simulink model "key_com_motor_ctrl"  (R2021a)
settings: configuration reference "f2_ctrl_config" (kept outside this file)
settings Model: DataDictionary=motor_data.sldd  Creator=Litao  LastModifiedBy=Litao
settings ConfigSetRef: SourceName=f2_ctrl_config

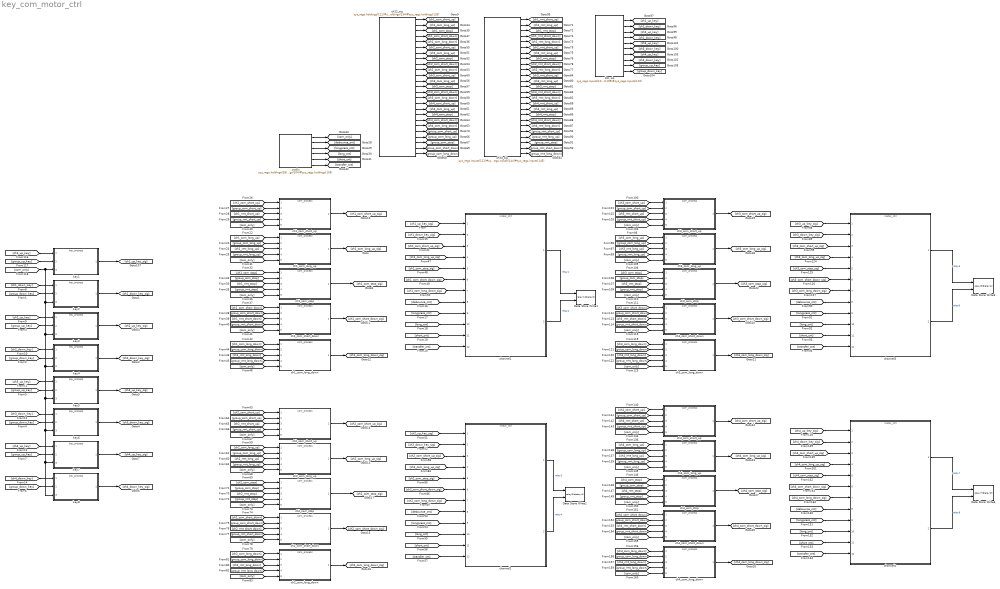
== system key_com_motor_ctrl ==
  Data Store Write1 : DataStoreWrite  DataStoreName=relay  DataStoreElements=relay(1)#relay(2)  IndexOptions=Index vector (dialog)  Indices=1  OutputSizes=1
  Data Store Write2 : DataStoreWrite  DataStoreName=relay  DataStoreElements=relay(3)#relay(4)  IndexOptions=Index vector (dialog)  Indices=1  OutputSizes=1
  Data Store Write3 : DataStoreWrite  DataStoreName=relay  DataStoreElements=relay(5)#relay(6)  IndexOptions=Index vector (dialog)  Indices=1  OutputSizes=1
  Data Store Write4 : DataStoreWrite  DataStoreName=relay  DataStoreElements=relay(7)#relay(8)  IndexOptions=Index vector (dialog)  Indices=1  OutputSizes=1
  btn_sig : DataStoreRead  DataStoreName=sys_regs  DataStoreElements=sys_regs.inputs(101)#sys_regs.inputs(102)#sys_regs.inputs(103)#sys_regs.inputs(104)#sys_regs.inputs(105)#sys_regs.inputs(106)#sys_regs.inputs(107)#sys_regs.inputs(108)#sys_regs.inputs(109)#sys_regs.inputs(110)  IndexOptions=Index vector (dialog)  Indices=1  OutputSizes=1
  ch12_sig : DataStoreRead  DataStoreName=sys_regs  DataStoreElements=sys_regs.holdings(111)#sys_regs.holdings(112)#sys_regs.holdings(113)#sys_regs.holdings(114)#sys_regs.holdings(115)#sys_regs.holdings(116)#sys_regs.holdings(117)#sys_regs.holdings(118)#sys_regs.holdings(119)#sys_regs.holdings(120)#sys_regs.holdings(121)#sys_regs.holdings(122)#sys_regs.holdings(123)#sys_regs.holdings(124)#sys_regs.holdings(125)#sys_regs.holdings(126)#sys_regs.holdings(127)#sys_regs.holdings(128)#sys_regs.holdings(129)#sys_regs.holdings(130)#sys_regs.holdings(131)#sys_regs.holdings(132)#sys_regs.holdings(133)#sys_regs.holdings(134)#sys_regs.holdings(135)  IndexOptions=Index vector (dialog)  Indices=1  OutputSizes=1
  ch1_com_long_down : ModelReference  ModelNameDialog=com_process.slx  SimulationMode=Normal  ModelReferenceVersion=1.8
  ch1_com_long_up : ModelReference  ModelNameDialog=com_process.slx  SimulationMode=Normal  ModelReferenceVersion=1.8
  ch1_com_short_down : ModelReference  ModelNameDialog=com_process.slx  SimulationMode=Normal  ModelReferenceVersion=1.8
  ch1_com_short_up : ModelReference  ModelNameDialog=com_process.slx  SimulationMode=Normal  ModelReferenceVersion=1.8
  ch1_com_stop : ModelReference  ModelNameDialog=com_process.slx  SimulationMode=Normal  ModelReferenceVersion=1.8
  ch2_com_long_down : ModelReference  ModelNameDialog=com_process.slx  SimulationMode=Normal  ModelReferenceVersion=1.8
  ch2_com_long_up : ModelReference  ModelNameDialog=com_process.slx  SimulationMode=Normal  ModelReferenceVersion=1.8
  ch2_com_short_down : ModelReference  ModelNameDialog=com_process.slx  SimulationMode=Normal  ModelReferenceVersion=1.8
  ch2_com_short_up : ModelReference  ModelNameDialog=com_process.slx  SimulationMode=Normal  ModelReferenceVersion=1.8
  ch2_com_stop : ModelReference  ModelNameDialog=com_process.slx  SimulationMode=Normal  ModelReferenceVersion=1.8
  ch34_sig : DataStoreRead  DataStoreName=sys_regs  DataStoreElements=sys_regs.inputs(121)#sys_regs.inputs(122)#sys_regs.inputs(123)#sys_regs.inputs(124)#sys_regs.inputs(125)#sys_regs.inputs(126)#sys_regs.inputs(127)#sys_regs.inputs(128)#sys_regs.inputs(129)#sys_regs.inputs(130)#sys_regs.inputs(131)#sys_regs.inputs(132)#sys_regs.inputs(133)#sys_regs.inputs(134)#sys_regs.inputs(135)#sys_regs.inputs(136)#sys_regs.inputs(137)#sys_regs.inputs(138)#sys_regs.inputs(139)#sys_regs.inputs(140)#sys_regs.inputs(141)#sys_regs.inputs(142)#sys_regs.inputs(143)#sys_regs.inputs(144)#sys_regs.inputs(145)  IndexOptions=Index vector (dialog)  Indices=1  OutputSizes=1
  ch3_com_long_down : ModelReference  ModelNameDialog=com_process.slx  SimulationMode=Normal  ModelReferenceVersion=1.8
  ch3_com_long_up : ModelReference  ModelNameDialog=com_process.slx  SimulationMode=Normal  ModelReferenceVersion=1.8
  ch3_com_short_down : ModelReference  ModelNameDialog=com_process.slx  SimulationMode=Normal  ModelReferenceVersion=1.8
  ch3_com_short_up : ModelReference  ModelNameDialog=com_process.slx  SimulationMode=Normal  ModelReferenceVersion=1.8
  ch3_com_stop : ModelReference  ModelNameDialog=com_process.slx  SimulationMode=Normal  ModelReferenceVersion=1.8
  ch4_com_long_down : ModelReference  ModelNameDialog=com_process.slx  SimulationMode=Normal  ModelReferenceVersion=1.8
  ch4_com_long_up : ModelReference  ModelNameDialog=com_process.slx  SimulationMode=Normal  ModelReferenceVersion=1.8
  ch4_com_short_down : ModelReference  ModelNameDialog=com_process.slx  SimulationMode=Normal  ModelReferenceVersion=1.8
  ch4_com_short_up : ModelReference  ModelNameDialog=com_process.slx  SimulationMode=Normal  ModelReferenceVersion=1.8
  ch4_com_stop : ModelReference  ModelNameDialog=com_process.slx  SimulationMode=Normal  ModelReferenceVersion=1.8
  channel{1..4} (4 alike) : ModelReference  ModelNameDialog=motor_ctrl.slx  SimulationMode=Normal  ModelReferenceVersion=1.19
  config : DataStoreRead  DataStoreName=sys_regs  DataStoreElements=sys_regs.holdings(38)#sys_regs.holdings(101)#sys_regs.holdings(102)#sys_regs.holdings(103)#sys_regs.holdings(104)#sys_regs.holdings(105)  IndexOptions=Index vector (dialog)  Indices=1  OutputSizes=1
  key{1..8} (8 alike) : ModelReference  ModelNameDialog=key_process.slx  SimulationMode=Normal  ModelReferenceVersion=1.7
  wires:
  config/1 -> [com_only]
  config/2 -> [debounce_cnt]
  config/3 -> [longpress_cnt]
  config/4 -> [long_cnt]
  config/5 -> [short_cnt]
  config/6 -> [transfer_cnt]
  ch12_sig/2 -> [ch1_com_long_up]
  ch12_sig/3 -> [ch1_com_stop]
  ch12_sig/4 -> [ch1_com_short_down]
  ch12_sig/5 -> [ch1_com_long_down]
  ch12_sig/6 -> [ch2_com_short_up]
  ch12_sig/7 -> [ch2_com_long_up]
  ch12_sig/8 -> [ch2_com_stop]
  ch12_sig/9 -> [ch2_com_short_down]
  ch12_sig/10 -> [ch2_com_long_down]
  ch12_sig/11 -> [ch3_com_short_up]
  ch12_sig/12 -> [ch3_com_long_up]
  ch12_sig/13 -> [ch3_com_stop]
  ch12_sig/14 -> [ch3_com_short_down]
  ch12_sig/15 -> [ch3_com_long_down]
  ch12_sig/16 -> [ch4_com_short_up]
  ch12_sig/17 -> [ch4_com_long_up]
  ch12_sig/18 -> [ch4_com_stop]
  ch12_sig/19 -> [ch4_com_short_down]
  ch12_sig/20 -> [ch4_com_long_down]
  ch12_sig/21 -> [group_com_short_up]
  ch34_sig/11 -> [ch3_rmt_short_up]
  ch34_sig/6 -> [ch2_rmt_short_up]
  ch34_sig/2 -> [ch1_rmt_long_up]
  ch34_sig/12 -> [ch3_rmt_long_up]
  ch34_sig/13 -> [ch3_rmt_stop]
  ch34_sig/1 -> [ch1_rmt_short_up]
  ch34_sig/14 -> [ch3_rmt_short_down]
  ch34_sig/20 -> [ch4_rmt_long_down]
  ch34_sig/16 -> [ch4_rmt_short_up]
  ch34_sig/18 -> [ch4_rmt_stop]
  ch34_sig/21 -> [group_rmt_short_up]
  ch34_sig/15 -> [ch3_rmt_long_down]
  ch34_sig/3 -> [ch1_rmt_stop]
  ch34_sig/17 -> [ch4_rmt_long_up]
  ch34_sig/8 -> [ch2_rmt_stop]
  ch34_sig/19 -> [ch4_rmt_short_down]
  ch34_sig/4 -> [ch1_rmt_short_down]
  ch34_sig/7 -> [ch2_rmt_long_up]
  ch34_sig/9 -> [ch2_rmt_short_down]
  ch34_sig/10 -> [ch2_rmt_long_down]
  ch34_sig/5 -> [ch1_rmt_long_down]
  ch12_sig/22 -> [group_com_long_up]
  ch12_sig/23 -> [group_com_stop]
  ch12_sig/24 -> [group_com_short_down]
  ch12_sig/25 -> [group_com_long_down]
  ch34_sig/22 -> [group_rmt_long_up]
  ch34_sig/23 -> [group_rmt_stop]
  ch34_sig/24 -> [group_rmt_short_down]
  ch34_sig/25 -> [group_rmt_long_down]
  btn_sig/1 -> [ch1_up_key]
  btn_sig/2 -> [ch1_down_key]
  btn_sig/3 -> [ch2_up_key]
  btn_sig/4 -> [ch2_down_key]
  btn_sig/5 -> [ch3_up_key]
  btn_sig/6 -> [ch3_down_key]
  btn_sig/7 -> [ch4_up_key]
  btn_sig/8 -> [ch4_down_key]
  btn_sig/9 -> [group_up_key]
  btn_sig/10 -> [group_down_key]
  [ch1_up_key] -> key1/1
  [group_up_key] -> key1/2
  [com_only] -> key8/3, key7/3, key6/3, key5/3, key4/3, key3/3, key2/3, key1/3
  key1/1 -> [ch1_up_key_sig]
  key2/1 -> [ch1_down_key_sig]
  key3/1 -> [ch2_up_key_sig]
  key4/1 -> [ch2_down_key_sig]
  key5/1 -> [ch3_up_key_sig]
  key6/1 -> [ch3_down_key_sig]
  key7/1 -> [ch4_up_key_sig]
  key8/1 -> [ch4_down_key_sig]
  [group_down_key] -> key2/2
  [group_down_key] -> key4/2
  [group_up_key] -> key3/2
  [group_down_key] -> key6/2
  [group_up_key] -> key5/2
  [group_down_key] -> key8/2
  [group_up_key] -> key7/2
  [ch1_down_key] -> key2/1
  [ch2_up_key] -> key3/1
  [ch2_down_key] -> key4/1
  [ch3_up_key] -> key5/1
  [ch3_down_key] -> key6/1
  [ch4_up_key] -> key7/1
  [ch4_down_key] -> key8/1
  [ch1_up_key_sig] -> channel1/1
  [ch1_down_key_sig] -> channel1/2
  [debounce_cnt] -> channel1/8
  [longpress_cnt] -> channel1/9
  [long_cnt] -> channel1/10
  [short_cnt] -> channel1/11
  [transfer_cnt] -> channel1/12
  [group_com_short_up] -> ch1_com_short_up/2
  [ch1_rmt_short_up] -> ch1_com_short_up/3
  [group_rmt_short_up] -> ch1_com_short_up/4
  [com_only] -> ch1_com_short_up/5
  ch1_com_short_up/1 -> [ch1_com_short_up_sig]
  [com_only] -> ch1_com_long_up/5
  [com_only] -> ch1_com_stop/5
  [com_only] -> ch1_com_short_down/5
  [com_only] -> ch1_com_long_down/5
  [ch1_com_long_up] -> ch1_com_long_up/1
  [group_com_long_up] -> ch1_com_long_up/2
  [ch1_rmt_long_up] -> ch1_com_long_up/3
  [group_rmt_long_up] -> ch1_com_long_up/4
  [ch1_com_stop] -> ch1_com_stop/1
  [group_com_stop] -> ch1_com_stop/2
  [ch1_rmt_stop] -> ch1_com_stop/3
  [group_rmt_stop] -> ch1_com_stop/4
  [ch1_com_short_down] -> ch1_com_short_down/1
  [group_com_short_down] -> ch1_com_short_down/2
  [ch1_rmt_short_down] -> ch1_com_short_down/3
  [group_rmt_short_down] -> ch1_com_short_down/4
  [ch1_com_long_down] -> ch1_com_long_down/1
  [group_com_long_down] -> ch1_com_long_down/2
  [ch1_rmt_long_down] -> ch1_com_long_down/3
  [group_rmt_long_down] -> ch1_com_long_down/4
  ch1_com_long_up/1 -> [ch1_com_long_up_sig]
  ch1_com_stop/1 -> [ch1_com_stop_sig]
  ch1_com_short_down/1 -> [ch1_com_short_down_sig]
  ch1_com_long_down/1 -> [ch1_com_long_down_sig]
  [ch1_com_short_up_sig] -> channel1/3
  [ch1_com_long_up_sig] -> channel1/4
  [ch1_com_stop_sig] -> channel1/5
  [ch1_com_long_down_sig] -> channel1/7
  [ch1_com_short_down_sig] -> channel1/6
  [group_rmt_long_up] -> ch2_com_long_up/4
  [com_only] -> ch2_com_short_up/5
  [ch2_rmt_stop] -> ch2_com_stop/3
  [ch2_rmt_short_up] -> ch2_com_short_up/3
  [ch2_com_stop_sig] -> channel2/5
  [ch2_com_long_up] -> ch2_com_long_up/1
  ch2_com_long_up/1 -> [ch2_com_long_up_sig]
  [ch2_com_long_down_sig] -> channel2/7
  [ch2_down_key_sig] -> channel2/2
  [longpress_cnt] -> channel2/9
  [group_rmt_short_up] -> ch2_com_short_up/4
  [group_com_short_up] -> ch2_com_short_up/2
  [ch2_com_long_up_sig] -> channel2/4
  [ch2_com_short_up] -> ch2_com_short_up/1
  [ch2_com_short_down] -> ch2_com_short_down/1
  [group_rmt_short_down] -> ch2_com_short_down/4
  ch2_com_short_up/1 -> [ch2_com_short_up_sig]
  [com_only] -> ch2_com_short_down/5
  [com_only] -> ch2_com_stop/5
  [ch2_rmt_short_down] -> ch2_com_short_down/3
  ch2_com_long_down/1 -> [ch2_com_long_down_sig]
  [group_com_short_down] -> ch2_com_short_down/2
  [ch2_com_stop] -> ch2_com_stop/1
  ch2_com_stop/1 -> [ch2_com_stop_sig]
  [transfer_cnt] -> channel2/12
  [ch2_com_short_up_sig] -> channel2/3
  [ch2_com_short_down_sig] -> channel2/6
  [ch2_rmt_long_down] -> ch2_com_long_down/3
  [group_rmt_long_down] -> ch2_com_long_down/4
  [group_rmt_stop] -> ch2_com_stop/4
  [com_only] -> ch2_com_long_up/5
  [group_com_stop] -> ch2_com_stop/2
  [short_cnt] -> channel2/11
  [group_com_long_up] -> ch2_com_long_up/2
  [debounce_cnt] -> channel2/8
  [ch2_up_key_sig] -> channel2/1
  [ch2_rmt_long_up] -> ch2_com_long_up/3
  [com_only] -> ch2_com_long_down/5
  [ch2_com_long_down] -> ch2_com_long_down/1
  ch2_com_short_down/1 -> [ch2_com_short_down_sig]
  [long_cnt] -> channel2/10
  [group_com_long_down] -> ch2_com_long_down/2
  [group_rmt_long_up] -> ch3_com_long_up/4
  [com_only] -> ch3_com_short_up/5
  [ch3_rmt_stop] -> ch3_com_stop/3
  [ch3_rmt_short_up] -> ch3_com_short_up/3
  [ch3_com_stop_sig] -> channel3/5
  [ch3_com_long_up] -> ch3_com_long_up/1
  ch3_com_long_up/1 -> [ch3_com_long_up_sig]
  [ch3_com_long_down_sig] -> channel3/7
  [ch3_down_key_sig] -> channel3/2
  [longpress_cnt] -> channel3/9
  [group_rmt_short_up] -> ch3_com_short_up/4
  [group_com_short_up] -> ch3_com_short_up/2
  [ch3_com_long_up_sig] -> channel3/4
  [ch3_com_short_up] -> ch3_com_short_up/1
  [ch3_com_short_down] -> ch3_com_short_down/1
  [group_rmt_short_down] -> ch3_com_short_down/4
  ch3_com_short_up/1 -> [ch3_com_short_up_sig]
  [com_only] -> ch3_com_short_down/5
  [com_only] -> ch3_com_stop/5
  [ch3_rmt_short_down] -> ch3_com_short_down/3
  ch3_com_long_down/1 -> [ch3_com_long_down_sig]
  [group_com_short_down] -> ch3_com_short_down/2
  [ch3_com_stop] -> ch3_com_stop/1
  ch3_com_stop/1 -> [ch3_com_stop_sig]
  [transfer_cnt] -> channel3/12
  [ch3_com_short_up_sig] -> channel3/3
  [ch3_com_short_down_sig] -> channel3/6
  [ch3_rmt_long_down] -> ch3_com_long_down/3
  [group_rmt_long_down] -> ch3_com_long_down/4
  [group_rmt_stop] -> ch3_com_stop/4
  [com_only] -> ch3_com_long_up/5
  [group_com_stop] -> ch3_com_stop/2
  [short_cnt] -> channel3/11
  [group_com_long_up] -> ch3_com_long_up/2
  [debounce_cnt] -> channel3/8
  [ch3_up_key_sig] -> channel3/1
  [ch3_rmt_long_up] -> ch3_com_long_up/3
  [com_only] -> ch3_com_long_down/5
  [ch3_com_long_down] -> ch3_com_long_down/1
  ch3_com_short_down/1 -> [ch3_com_short_down_sig]
  [long_cnt] -> channel3/10
  [group_com_long_down] -> ch3_com_long_down/2
  [group_rmt_long_up] -> ch4_com_long_up/4
  [com_only] -> ch4_com_short_up/5
  [ch4_rmt_stop] -> ch4_com_stop/3
  [ch4_rmt_short_up] -> ch4_com_short_up/3
  [ch4_com_stop_sig] -> channel4/5
  [ch4_com_long_up] -> ch4_com_long_up/1
  ch4_com_long_up/1 -> [ch4_com_long_up_sig]
  [ch4_com_long_down_sig] -> channel4/7
  [ch4_down_key_sig] -> channel4/2
  [longpress_cnt] -> channel4/9
  [group_rmt_short_up] -> ch4_com_short_up/4
  [group_com_short_up] -> ch4_com_short_up/2
  [ch4_com_long_up_sig] -> channel4/4
  [ch4_com_short_up] -> ch4_com_short_up/1
  [ch4_com_short_down] -> ch4_com_short_down/1
  [group_rmt_short_down] -> ch4_com_short_down/4
  ch4_com_short_up/1 -> [ch4_com_short_up_sig]
  [com_only] -> ch4_com_short_down/5
  [com_only] -> ch4_com_stop/5
  [ch4_rmt_short_down] -> ch4_com_short_down/3
  ch4_com_long_down/1 -> [ch4_com_long_down_sig]
  [group_com_short_down] -> ch4_com_short_down/2
  [ch4_com_stop] -> ch4_com_stop/1
  ch4_com_stop/1 -> [ch4_com_stop_sig]
  [transfer_cnt] -> channel4/12
  [ch4_com_short_up_sig] -> channel4/3
  [ch4_com_short_down_sig] -> channel4/6
  [ch4_rmt_long_down] -> ch4_com_long_down/3
  [group_rmt_long_down] -> ch4_com_long_down/4
  [group_rmt_stop] -> ch4_com_stop/4
  [com_only] -> ch4_com_long_up/5
  [group_com_stop] -> ch4_com_stop/2
  [short_cnt] -> channel4/11
  [group_com_long_up] -> ch4_com_long_up/2
  [debounce_cnt] -> channel4/8
  [ch4_up_key_sig] -> channel4/1
  [ch4_rmt_long_up] -> ch4_com_long_up/3
  [com_only] -> ch4_com_long_down/5
  [ch4_com_long_down] -> ch4_com_long_down/1
  ch4_com_short_down/1 -> [ch4_com_short_down_sig]
  [long_cnt] -> channel4/10
  [group_com_long_down] -> ch4_com_long_down/2
  [ch1_com_short_up] -> ch1_com_short_up/1
  ch12_sig/1 -> [ch1_com_short_up]
  channel1/1 -> Data Store Write1/1  "relay1"
  channel1/2 -> Data Store Write1/2  "relay2"
  channel2/1 -> Data Store Write2/1  "relay3"
  channel2/2 -> Data Store Write2/2  "relay4"
  channel3/1 -> Data Store Write3/1  "relay5"
  channel3/2 -> Data Store Write3/2  "relay6"
  channel4/1 -> Data Store Write4/1  "relay7"
  channel4/2 -> Data Store Write4/2  "relay8"
